simulink model "Car_Following_Test"  (R2020b)
settings: Solver=FixedStepAuto  StartTime=0.0  StopTime=120  FixedStep=0.05  RelTol=1e-3
libraries: SignalEditorBlockLib x1
settings Model: Creator=duanx  LastModifiedBy=duanx

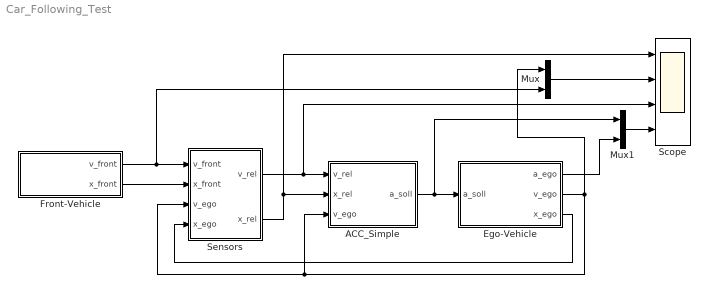
== system Car_Following_Test ==
  ACC_Simple : Subsystem
  Ego-Vehicle : Subsystem
  Front-Vehicle : Subsystem
  Mux : Mux  Inputs=2
  Mux1 : Mux  Inputs=2
  Scope : Scope  NumInputPorts=4
  Sensors : Subsystem
  wires:
  Front-Vehicle/1(v_front) -> Mux/2, Sensors/1(v_front)
  Front-Vehicle/2(x_front) -> Sensors/2(x_front)
  Ego-Vehicle/2(v_ego) -> ACC_Simple/3(v_ego), Sensors/3(v_ego), Mux/1
  Ego-Vehicle/3(x_ego) -> Sensors/4(x_ego)
  Sensors/1(v_rel) -> Scope/3, ACC_Simple/1(v_rel)
  Sensors/2(x_rel) -> Scope/1, ACC_Simple/2(x_rel)
  ACC_Simple/1(a_soll) -> Mux1/1, Ego-Vehicle/1(a_soll)
  Mux/1 -> Scope/2
  Ego-Vehicle/1(a_ego) -> Mux1/2
  Mux1/1 -> Scope/4

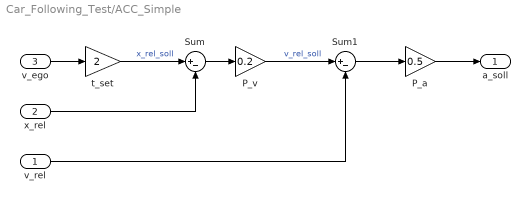
== system Car_Following_Test/ACC_Simple ==
  v_rel : Inport  Unit=m/s
  x_rel : Inport  Port=2  Unit=m
  v_ego : Inport  Port=3  Unit=m/s
  P_a : Gain  Gain=0.5
  P_v : Gain  Gain=0.2
  Sum : Sum  Inputs=|+-
  Sum1 : Sum  Inputs=|+-
  t_set : Gain  Gain=2
  a_soll : Outport
  wires:
  v_ego/1 -> t_set/1
  Sum/1 -> P_v/1
  x_rel/1 -> Sum/2
  t_set/1 -> Sum/1  "x_rel_soll"
  Sum1/1 -> P_a/1
  P_v/1 -> Sum1/1  "v_rel_soll"
  v_rel/1 -> Sum1/2
  P_a/1 -> a_soll/1

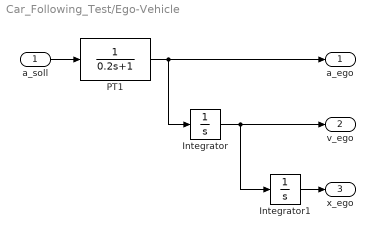
== system Car_Following_Test/Ego-Vehicle ==
  a_soll : Inport
  Integrator : Integrator
  Integrator1 : Integrator
  PT1 : TransferFcn  Denominator=[0.2 1]
  a_ego : Outport
  v_ego : Outport  Port=2
  x_ego : Outport  Port=3
  wires:
  a_soll/1 -> PT1/1
  PT1/1 -> Integrator/1, a_ego/1
  Integrator/1 -> v_ego/1, Integrator1/1
  Integrator1/1 -> x_ego/1

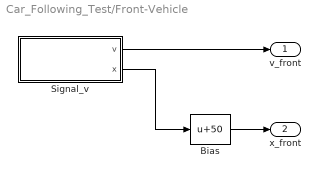
== system Car_Following_Test/Front-Vehicle ==
  Bias : Bias  Bias=50
  Signal_v : Subsystem
  v_front : Outport  Unit=m/s
  x_front : Outport  Port=2  Unit=m
  wires:
  Bias/1 -> x_front/1
  Signal_v/1(v) -> v_front/1
  Signal_v/2(x) -> Bias/1

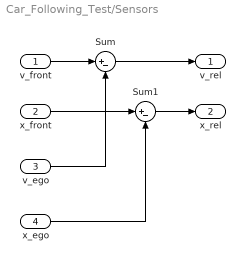
== system Car_Following_Test/Sensors ==
  v_front : Inport  Unit=m/s
  x_front : Inport  Port=2  Unit=m
  v_ego : Inport  Port=3  Unit=m/s
  x_ego : Inport  Port=4  Unit=m
  Sum : Sum  Inputs=|+-
  Sum1 : Sum  Inputs=|+-
  v_rel : Outport
  x_rel : Outport  Port=2
  wires:
  Sum1/1 -> x_rel/1
  Sum/1 -> v_rel/1
  v_front/1 -> Sum/1
  v_ego/1 -> Sum/2
  x_front/1 -> Sum1/1
  x_ego/1 -> Sum1/2

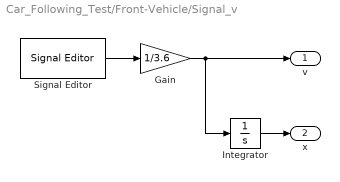
== system Car_Following_Test/Front-Vehicle/Signal_v ==
  Gain : Gain  Gain=1/3.6
  Integrator : Integrator
  Signal Editor : SignalEditorBlockLib/Signal Editor  FileName=Signal_v_profile.mat  ActiveScenario=const_v  ActiveSignal=v  IsBus=off  OutputBusObjectStr=Bus: BusObject  SampleTime=0  Interpolate=off  ZeroCross=off  OutputAfterFinalValue=Setting to zero  Unit=inherit  PreserveSignalName=on
  v : Outport  Unit=m/s
  x : Outport  Port=2  Unit=m
  wires:
  Integrator/1 -> x/1
  Signal Editor/1 -> Gain/1
  Gain/1 -> Integrator/1, v/1
